simulink model "My_Template"  (R2022b)
settings: Solver=VariableStepAuto  StartTime=0.0  StopTime=10.0  RelTol=1e-3
undefined symbols (not defined in the file): x0
settings Model: Creator=user  LastModifiedBy=user

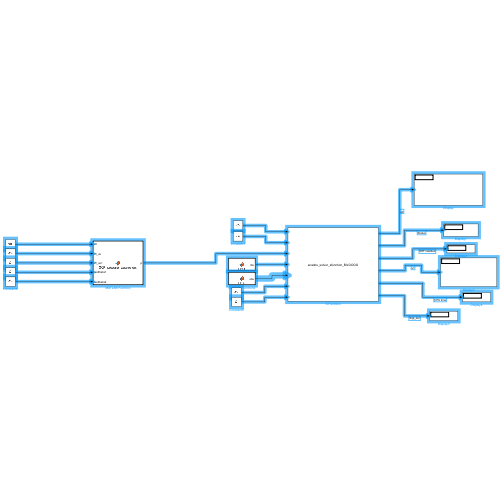
[thumbnail: Simulink's stored preview of the top-level diagram]
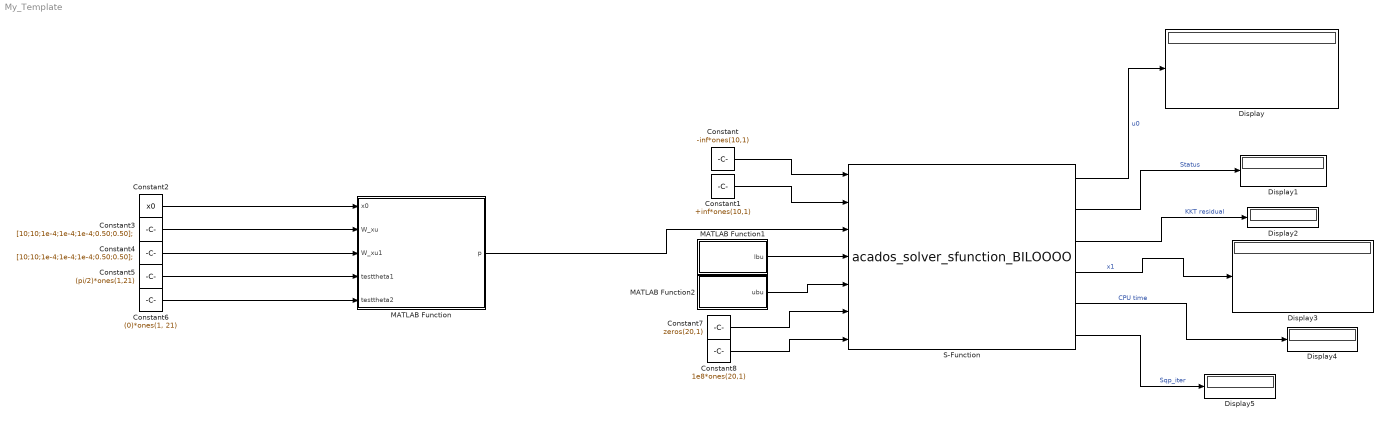
== system My_Template ==
  Constant : Constant  Value=-inf*ones(10,1)
  Constant1 : Constant  Value=+inf*ones(10,1)
  Constant2 : Constant  Value=x0
  Constant3 : Constant  Value=[10;10;1e-4;1e-4;1e-4;0.50;0.50];
  Constant4 : Constant  Value=[10;10;1e-4;1e-4;1e-4;0.50;0.50];
  Constant5 : Constant  Value=(pi/2)*ones(1,21)
  Constant6 : Constant  Value=(0)*ones(1, 21)
  Constant7 : Constant  Value=zeros(20,1)
  Constant8 : Constant  Value=1e8*ones(20,1)
  Display{,1..5} (6 alike) : Display
  MATLAB Function : MATLAB Function  TreatAsAtomicUnit=on
  MATLAB Function1 : MATLAB Function  TreatAsAtomicUnit=on
  MATLAB Function2 : MATLAB Function  TreatAsAtomicUnit=on
  S-Function : S-Function  FunctionName=acados_solver_sfunction_BILOOOO  SFunctionDeploymentMode=off  EnableBusSupport=off
  wires:
  MATLAB Function1/1(lbu) -> S-Function/4
  S-Function/4 -> Display3/1  "x1"
  S-Function/2 -> Display1/1  "Status"
  Constant3/1 -> MATLAB Function/2(W_xu)
  MATLAB Function/1(p) -> S-Function/3
  S-Function/1 -> Display/1  "u0"
  Constant8/1 -> S-Function/7
  S-Function/3 -> Display2/1  "KKT residual"
  Constant2/1 -> MATLAB Function/1(x0)
  Constant1/1 -> S-Function/2
  Constant/1 -> S-Function/1
  Constant7/1 -> S-Function/6
  S-Function/5 -> Display4/1  "CPU time"
  S-Function/6 -> Display5/1  "Sqp_iter"
  Constant4/1 -> MATLAB Function/3(W_xu1)
  Constant5/1 -> MATLAB Function/4(testtheta1)
  Constant6/1 -> MATLAB Function/5(testtheta2)
  MATLAB Function2/1(ubu) -> S-Function/5

== matlab function My_Template/MATLAB Function1 ==
  data: lbu output
function lbu = LBU
% Define lower bounds for control inputs
lbu_control = [-11.5; -1; -11.5; -1]; % Control inputs

% Determine how many times to repeat the control bounds
num_repeats = ceil(80 / length(lbu_control)); % Calculate how many times to repeat
lbu = repmat(lbu_control, num_repeats, 1); % Repeat to create a long enough array
lbu = lbu(1:80); % Truncate to exactly 80 elements

% Check size
assert(length(lbu) == 80, 'Lower bounds array must have 80 elements.');

end

== matlab function My_Template/MATLAB Function ==
  data: x0 input; p output; W_xu input; W_xu1 input; testtheta1 input; testtheta2 input
function p = OCP_prepare_parameters(x0, W_xu, W_xu1, testtheta1, testtheta2)
    nx = length(x0);
    nu = 4;
    ocp_N = 20; % Number of prediction steps
    % Initialize the parameter array
    p = zeros(504, 1); % 504 elements as per your structure
    D1=W2_newnew(x0);D2=W3_newnew(x0); %% referencing    
    % Prepare reference points
    current_state1 = x0(1:2); % Use the updated x0
    current_state2 = x0(6:7);
    
    closest_idx1 = findClosestPoint(current_state1, D1);
    closest_idx2 = findClosestPoint(current_state2, D2);
    
    % Reference points for car 1
    if closest_idx1 + ocp_N <= size(D1, 2)
        reference_points1 = D1(:, closest_idx1:closest_idx1+ocp_N);
    else
        remaining_points1 = size(D1, 2) - closest_idx1 + 1;
        reference_points1 = D1(:, closest_idx1:end);
        additional_points1 = (ocp_N + 1) - remaining_points1;
        
        last_x1 = D1(1, end);
        last_y1 = D1(2, end);
        new_x1 = last_x1 - (1:additional_points1) * 0.1; % Assuming 0.1m per step
        new_y1 = last_y1 * ones(1, additional_points1);
        
        extended_points1 = [new_x1; new_y1];
        reference_points1 = [reference_points1, extended_points1];
    end
    
    % Reference points for car 2
    if closest_idx2 + ocp_N <= size(D2, 2)
        reference_points2 = D2(:, closest_idx2:closest_idx2+ocp_N);
    else
        remaining_points2 = size(D2, 2) - closest_idx2 + 1;
        reference_points2 = D2(:, closest_idx2:end);
        additional_points2 = (ocp_N + 1) - remaining_points2;

        last_x2 = D2(1, end);
        last_y2 = D2(2, end);
        new_x2 = last_x2 + (1:additional_points2) * 0.1; % Assuming 0.1m per step
        new_y2 = last_y2 * ones(1, additional_points2);
        
        extended_points2 = [new_x2; new_y2];
        reference_points2 = [reference_points2, extended_points2];
    end
    
    % Combine reference points and prepare parameter vector
    x_traj_init = [reference_points1; testtheta1'; zeros(1, ocp_N + 1); zeros(1, ocp_N + 1); ...
                   reference_points2; testtheta2'; zeros(1, ocp_N + 1); zeros(1, ocp_N + 1)];
    
    % Fill the parameter array
    for jj = 1:ocp_N
        p((jj - 1) * nx + 1:jj * nx) = x_traj_init(:, jj);
    end
    
    % Weights - example, adapt as needed
    p(nx*ocp_N + 1:nx*ocp_N + 14) = [W_xu1(1:5); W_xu(1:5); W_xu1(6:7); W_xu(6:7)];

    % Check if the size of p is correct
    assert(length(p) == 504, 'Parameter array must have 504 elements.');

    % Output parameter array
end

== matlab function My_Template/MATLAB Function2 ==
  data: ubu output
function ubu = UBU
% Define lower bounds for control inputs
ubu_control = [+11.5; 1; 11.5; 1]; % Control inputs

% Determine how many times to repeat the control bounds
num_repeats = ceil(80 / length(ubu_control)); % Calculate how many times to repeat
ubu = repmat(ubu_control, num_repeats, 1); % Repeat to create a long enough array
ubu = ubu(1:80); % Truncate to exactly 80 elements

% Check size
assert(length(ubu) == 80, 'Lower bounds array must have 80 elements.');

end
